simulink model "VM_Ctrl_V1"  (R2018a)
settings: Solver=VariableStepAuto  StartTime=0.0  StopTime=10.0  FixedStep=sampletime  RelTol=1e-3  EnableMultiTasking=on
PreLoadFcn:
  | VM_Ctrl_V1_BusInfo
libraries: simulink x2
settings Model: Creator=IAEC nishito  LastModifiedBy=nishito
settings DataIOCC: LimitDataPoints=on  SaveFormat=Array  SignalLoggingSaveFormat=ModelDataLogs  SaveOutput=off
settings OptimizationCC: DefaultParameterBehavior=Inlined  ExpressionDepthLimit=2147483647  LifeSpan=inf
settings DebuggingCC: UnderspecifiedInitializationDetection=Classic  MergeDetectMultiDrivingBlocksExec=none  SolverPrmCheckMsg=warning  FcnCallInpInsideContextMsg=warning  StateNameClashWarn=warning  SFUnexpectedBacktrackingDiag=warning  SFNoUnconditionalDefaultTransitionDiag=warning  SFExecutionAtInitializationDiag=none
settings HardwareCC: ProdBitPerPointer=32  ProdBitPerSizeT=32  ProdBitPerPtrDiffT=32  ProdLargestAtomicFloat=None  ProdIntDivRoundTo=Undefined  ProdEndianess=Unspecified  ProdWordSize=32  ProdHWDeviceType=32-bit Generic
settings ModelReferenceCC: UpdateModelReferenceTargets=IfOutOfDate  PropagateSignalLabelsOutOfModel=off
settings CodeAppCC: StateflowObjectComments=on
settings GRTTargetCC: TargetLangStandard=C89/C90 (ANSI)  GeneratePreprocessorConditionals=Disable all  CombineOutputUpdateFcns=off  GRTInterface=on
settings ConfigComp: CovMetricSettings=dw  CovHtmlReporting=on  CovSaveCumulativeToWorkspaceVar=on  CovSaveSingleToWorkspaceVar=on  CovExternalEMLEnable=off

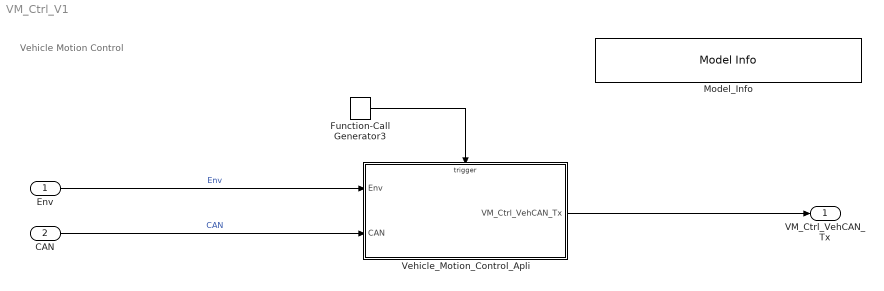
== system VM_Ctrl_V1 ==
  note: Vehicle Motion Control
  Env : Inport  OutDataTypeStr=Bus: Environment_Bus
      settings: AttributesFormatString=<%<OutDataTypeStr>>
  CAN : Inport  Port=2  OutDataTypeStr=Bus: CAN_Bus
      settings: AttributesFormatString=<%<OutDataTypeStr>>
  Function-Call Generator3 : simulink/Ports & Subsystems/Function-Call Generator  sample_time=0.05  numberOfIterations=1
      settings: AttributesFormatString=<sample_time=%<sample_time>>
  Model_Info : simulink/Model-Wide Utilities/Model Info  Frame=on  DisplayStringWithTags=|  HorizontalTextAlignment=Left  LeftAlignmentValue=0.02
      | Version  %<ModelVersion>
      | LastModifided by %<LastModifiedBy>  Date %<LastModificationDate>
      | Description  %<Description>
  Vehicle_Motion_Control_Apli : Subsystem
  VM_Ctrl_VehCAN_Tx : Outport  OutDataTypeStr=Bus: VM_Ctrl_VehCAN_Tx_Bus
      settings: AttributesFormatString=<%<OutDataTypeStr>>
  wires:
  Vehicle_Motion_Control_Apli/1(VM_Ctrl_VehCAN_Tx) -> VM_Ctrl_VehCAN_Tx/1
  CAN/1 -> Vehicle_Motion_Control_Apli/2(CAN)  "CAN"
  Env/1 -> Vehicle_Motion_Control_Apli/1(Env)  "Env"
  Function-Call Generator3/1 -> Vehicle_Motion_Control_Apli/Trigger

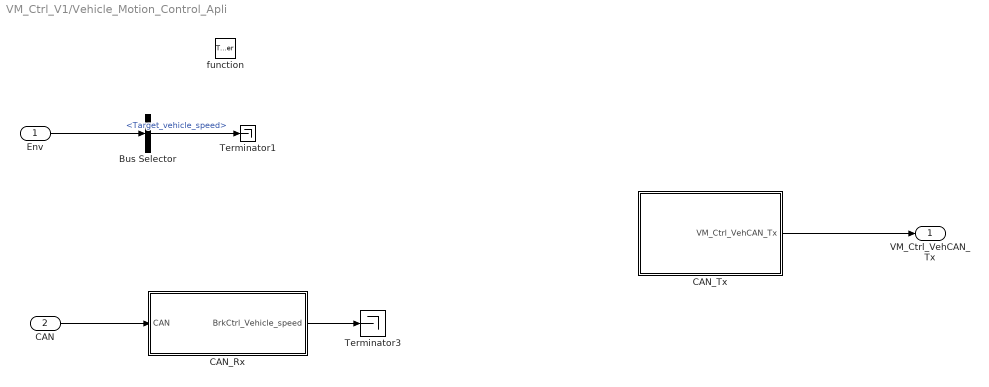
== system VM_Ctrl_V1/Vehicle_Motion_Control_Apli ==
  Env : Inport
  CAN : Inport  Port=2
  function : TriggerPort  TriggerType=function-call  VariantControl=Variant
  Bus Selector : BusSelector  OutputSignals=Target_vehicle_speed
  CAN_Rx : Subsystem
  CAN_Tx : Subsystem
  Terminator1 : Terminator
  Terminator3 : Terminator
  VM_Ctrl_VehCAN_Tx : Outport
  wires:
  Env/1 -> Bus Selector/1
  CAN/1 -> CAN_Rx/1(CAN)
  Bus Selector/1 -> Terminator1/1  "<Target_vehicle_speed>"
  CAN_Rx/1(BrkCtrl_Vehicle_speed) -> Terminator3/1
  CAN_Tx/1(VM_Ctrl_VehCAN_Tx) -> VM_Ctrl_VehCAN_Tx/1

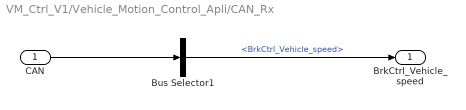
== system VM_Ctrl_V1/Vehicle_Motion_Control_Apli/CAN_Rx ==
  CAN : Inport
  Bus Selector1 : BusSelector  OutputSignals=VehCAN.BrakeCtrl_VehCAN_Tx.BrkCtrl_Vehicle_speed
  BrkCtrl_Vehicle_speed : Outport
  wires:
  Bus Selector1/1 -> BrkCtrl_Vehicle_speed/1  "<BrkCtrl_Vehicle_speed>"
  CAN/1 -> Bus Selector1/1

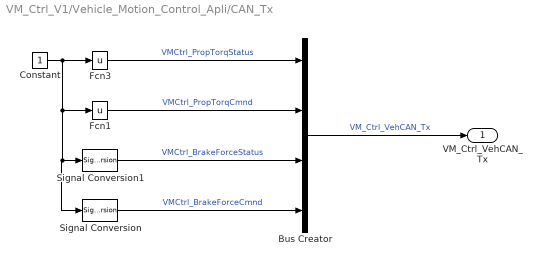
== system VM_Ctrl_V1/Vehicle_Motion_Control_Apli/CAN_Tx ==
  Bus Creator : BusCreator  Inputs=4  OutDataTypeStr=Bus: VM_Ctrl_VehCAN_Tx_Bus
      settings: AttributesFormatString=<%<OutDataTypeStr>>
  Constant : Constant
  Fcn1 : Fcn  Expr=u
  Fcn3 : Fcn  Expr=u
  Signal Conversion : SignalConversion  OverrideOpt=off
  Signal Conversion1 : SignalConversion  OverrideOpt=off
  VM_Ctrl_VehCAN_Tx : Outport
  wires:
  Fcn3/1 -> Bus Creator/1  "VMCtrl_PropTorqStatus"
  Constant/1 -> Fcn1/1, Signal Conversion/1, Signal Conversion1/1, Fcn3/1
  Fcn1/1 -> Bus Creator/2  "VMCtrl_PropTorqCmnd"
  Bus Creator/1 -> VM_Ctrl_VehCAN_Tx/1  "VM_Ctrl_VehCAN_Tx"
  Signal Conversion1/1 -> Bus Creator/3  "VMCtrl_BrakeForceStatus"
  Signal Conversion/1 -> Bus Creator/4  "VMCtrl_BrakeForceCmnd"
